simulink library "ammclib_bam_s32k14x"  (Simulink 9.0)
settings: Solver=ode45  StartTime=0.0  StopTime=10.0  RelTol=1e-3
undefined symbols (not defined in the file): f16A1, f16A2, f16B0, f16B1, f16B2, f16C1, f16CC1, f16CC1sc, f16CC1sc_D, f16CC1sc_Q, f16CC1scD, f16CC1scQ, f16CC2, f16CC2sc, f16CC2sc_D, f16CC2sc_Q, f16CC2scD, f16CC2scQ, f16DerivGain, f16EGain, f16FiltCoef, f16HystOff, f16HystOn, f16IGain, f16IntegGain, f16IntegGainFW, f16IntegGainQ, f16Kd, f16Kq, f16Limit, f16LowerLim, f16LowerLimit_D, f16LowerLimit_Q, f16ModIndex, f16OutValOff, f16OutValOn, f16PropGain, f16PropGainFW, f16PropGainQ, f16RampDown, f16RampUp, f16UGain, f16UpperLim, f16UpperLimit, f16UpperLimit_D, f16UpperLimit_Q, f16WIGain, f32A1, f32A2, f32B0, f32B1, f32B2, f32C1, f32CC1, f32CC1sc, f32CC1sc_D, f32CC1sc_Q, f32CC1scD, f32CC1scQ, f32CC2 ... (+122)
(part 8 of 11)

== system ammclib_bam_s32k14x/GMCLIB/bam_f32/GMCLIB_ClarkInv_F32 ==
  note: ---------------------------------------------------------------------------------------------------------------------------------------------------------------------------------------------------
  f32Alpha : Inport
  f32Beta : Inport  Port=2
  GMCLIB_ClarkInv_SF_F32 : S-Function  FunctionName=GMCLIB_ClarkInv_SF_F32  SFunctionDeploymentMode=off  EnableBusSupport=off
  copyright : Subsystem
      mask Display:
      | text(10,90,'FILE:');text(10,75,'DESRIPTION:')
      | text(10,60,'COPYRIGHT:')
      | text(10,45,'VERSION:')
      | text(10,30,'DATE:')
  copyright2 : Subsystem
      mask Display:
      | text(10,90,'GMCLIB_ClarkInv_BAM_F32.mdl');text(10,75,'Inverse Clarke transformation');text(10,60,'NXP')
      | text(10,45,'0.1');text(10,30,'30-Aug-2011');
  logo : Subsystem
      mask Display: image(imread('logo.jpg'))
  f32A : Outport
  f32B : Outport  Port=2
  f32C : Outport  Port=3
  wires:
  GMCLIB_ClarkInv_SF_F32/3 -> f32C/1
  GMCLIB_ClarkInv_SF_F32/2 -> f32B/1
  GMCLIB_ClarkInv_SF_F32/1 -> f32A/1
  f32Beta/1 -> GMCLIB_ClarkInv_SF_F32/2
  f32Alpha/1 -> GMCLIB_ClarkInv_SF_F32/1

== system ammclib_bam_s32k14x/GMCLIB/bam_f32/GMCLIB_Clark_F32 ==
  note: ---------------------------------------------------------------------------------------------------------------------------------------------------------------------------------------------------
  f32A : Inport
  f32B : Inport  Port=2
  f32C : Inport  Port=3
  GMCLIB_Clark_SF_F32 : S-Function  FunctionName=GMCLIB_Clark_SF_F32  SFunctionDeploymentMode=off  EnableBusSupport=off
  copyright : Subsystem
      mask Display:
      | text(10,90,'FILE:');text(10,75,'DESRIPTION:')
      | text(10,60,'COPYRIGHT:')
      | text(10,45,'VERSION:')
      | text(10,30,'DATE:')
  copyright2 : Subsystem
      mask Display:
      | text(10,90,'GMCLIB_Clark_BAM_F32.mdl');text(10,75,'Clarke transformation.');text(10,60,'NXP')
      | text(10,45,'0.1');text(10,30,'29-Aug-2011');
  logo : Subsystem
      mask Display: image(imread('logo.jpg'))
  f32Alpha : Outport
  f32Beta : Outport  Port=2
  wires:
  GMCLIB_Clark_SF_F32/2 -> f32Beta/1
  GMCLIB_Clark_SF_F32/1 -> f32Alpha/1
  f32C/1 -> GMCLIB_Clark_SF_F32/3
  f32B/1 -> GMCLIB_Clark_SF_F32/2
  f32A/1 -> GMCLIB_Clark_SF_F32/1

== system ammclib_bam_s32k14x/GMCLIB/bam_f32/GMCLIB_DecouplingPMSM_F32 ==
  note: ---------------------------------------------------------------------------------------------------------------------------------------------------------------------------------------------------
  f32Ud : Inport
  f32Uq : Inport  Port=2
  f32Id : Inport  Port=3
  f32Iq : Inport  Port=4
  f32AngVel : Inport  Port=5
  GMCLIB_DecouplingPMSM_SF_F32 : S-Function  FunctionName=GMCLIB_DecouplingPMSM_SF_F32  Parameters=f32Kd,s16KdShift,f32Kq,s16KqShift  SFunctionDeploymentMode=off  EnableBusSupport=off
  copyright : Subsystem
      mask Display:
      | text(10,90,'FILE:');text(10,75,'DESRIPTION:')
      | text(10,60,'COPYRIGHT:')
      | text(10,45,'VERSION:')
      | text(10,30,'DATE:')
  copyright2 : Subsystem
      mask Display:
      | text(10,90,'GMCLIB_DecouplingPMSM_BAM_F32.mdl');text(10,75,'Decoupling of d and q axis of PMSM model.');text(10,60,'NXP')
      | text(10,45,'0.1');text(10,30,'14-Sep-2011');
  logo : Subsystem
      mask Display: image(imread('logo.jpg'))
  f32UdDec : Outport
  f32UqDec : Outport  Port=2
  wires:
  GMCLIB_DecouplingPMSM_SF_F32/2 -> f32UqDec/1
  GMCLIB_DecouplingPMSM_SF_F32/1 -> f32UdDec/1
  f32AngVel/1 -> GMCLIB_DecouplingPMSM_SF_F32/5
  f32Iq/1 -> GMCLIB_DecouplingPMSM_SF_F32/4
  f32Id/1 -> GMCLIB_DecouplingPMSM_SF_F32/3
  f32Uq/1 -> GMCLIB_DecouplingPMSM_SF_F32/2
  f32Ud/1 -> GMCLIB_DecouplingPMSM_SF_F32/1

== system ammclib_bam_s32k14x/GMCLIB/bam_f32/GMCLIB_ElimDcBusRip_F32 ==
  note: ---------------------------------------------------------------------------------------------------------------------------------------------------------------------------------------------------
  f32Alpha : Inport
  f32Beta : Inport  Port=2
  f32ArgDcBusMsr : Inport  Port=3
  GMCLIB_ElimDcBusRip_SF : S-Function  FunctionName=GMCLIB_ElimDcBusRip_SF_F32  Parameters=f32ModIndex  SFunctionDeploymentMode=off  EnableBusSupport=off
  copyright : Subsystem
      mask Display: text(10,90,'FILE:');text(10,75,'DESRIPTION:');text(10,60,'COPYRIGHT:');text(10,45,'VERSION:');text(10,30,'DATE:')
  copyright2 : Subsystem
      mask Display: text(10,90,'GMCLIB_ElimDcBusRip_BAM_F32.mdl');text(10,75,'DC Bus voltage ripple elimination function.');text(10,60,'NXP');text(10,45,'0.1');text(10,30,'12-Jun-2015');
  logo : Subsystem
      mask Display: image(imread('logo.jpg'))
  f32AlphaOut : Outport
  f32BetaOut : Outport  Port=2
  wires:
  GMCLIB_ElimDcBusRip_SF/2 -> f32BetaOut/1
  GMCLIB_ElimDcBusRip_SF/1 -> f32AlphaOut/1
  f32ArgDcBusMsr/1 -> GMCLIB_ElimDcBusRip_SF/3
  f32Beta/1 -> GMCLIB_ElimDcBusRip_SF/2
  f32Alpha/1 -> GMCLIB_ElimDcBusRip_SF/1

== system ammclib_bam_s32k14x/GMCLIB/bam_f32/GMCLIB_ParkInv_F32 ==
  note: ---------------------------------------------------------------------------------------------------------------------------------------------------------------------------------------------------
  f32D : Inport
  f32Q : Inport  Port=2
  f32Sin : Inport  Port=3
  f32Cos : Inport  Port=4
  GMCLIB_ParkInv_SF : S-Function  FunctionName=GMCLIB_ParkInv_SF_F32  SFunctionDeploymentMode=off  EnableBusSupport=off
  copyright : Subsystem
      mask Display:
      | text(10,90,'FILE:');text(10,75,'DESRIPTION:')
      | text(10,60,'COPYRIGHT:')
      | text(10,45,'VERSION:')
      | text(10,30,'DATE:')
  copyright2 : Subsystem
      mask Display:
      | text(10,90,'GMCLIB_ParkInv_BAM_F32.mdl');text(10,75,'Inverse Park transformation.');text(10,60,'Freescale')
      | text(10,45,'0.1');text(10,30,'19-Sep-2011');
  logo : Subsystem
      mask Display: image(imread('logo.jpg'))
  f32Alpha : Outport
  f32Beta : Outport  Port=2
  wires:
  GMCLIB_ParkInv_SF/2 -> f32Beta/1
  GMCLIB_ParkInv_SF/1 -> f32Alpha/1
  f32Cos/1 -> GMCLIB_ParkInv_SF/4
  f32Sin/1 -> GMCLIB_ParkInv_SF/3
  f32Q/1 -> GMCLIB_ParkInv_SF/2
  f32D/1 -> GMCLIB_ParkInv_SF/1

== system ammclib_bam_s32k14x/GMCLIB/bam_f32/GMCLIB_Park_F32 ==
  note: ---------------------------------------------------------------------------------------------------------------------------------------------------------------------------------------------------
  f32Alpha : Inport
  f32Beta : Inport  Port=2
  f32Sin : Inport  Port=3
  f32Cos : Inport  Port=4
  GMCLIB_Park_SF : S-Function  FunctionName=GMCLIB_Park_SF_F32  SFunctionDeploymentMode=off  EnableBusSupport=off
  copyright : Subsystem
      mask Display:
      | text(10,90,'FILE:');text(10,75,'DESRIPTION:')
      | text(10,60,'COPYRIGHT:')
      | text(10,45,'VERSION:')
      | text(10,30,'DATE:')
  copyright2 : Subsystem
      mask Display:
      | text(10,90,'GMCLIB_Park_BAM_F32.mdl');text(10,75,'Park transformation.');text(10,60,'NXP')
      | text(10,45,'0.1');text(10,30,'19-Sep-2011');
  logo : Subsystem
      mask Display: image(imread('logo.jpg'))
  f32D : Outport
  f32Q : Outport  Port=2
  wires:
  GMCLIB_Park_SF/2 -> f32Q/1
  GMCLIB_Park_SF/1 -> f32D/1
  f32Cos/1 -> GMCLIB_Park_SF/4
  f32Sin/1 -> GMCLIB_Park_SF/3
  f32Beta/1 -> GMCLIB_Park_SF/2
  f32Alpha/1 -> GMCLIB_Park_SF/1

== system ammclib_bam_s32k14x/GMCLIB/bam_f32/GMCLIB_PwmIct_F32 ==
  note: ---------------------------------------------------------------------------------------------------------------------------------------------------------------------------------------------------
  f32In1 : Inport
  f32In2 : Inport  Port=2
  GMCLIB_PwmIct_SF : S-Function  FunctionName=GMCLIB_PwmIct_SF_F32  SFunctionDeploymentMode=off  EnableBusSupport=off
  copyright : Subsystem
      mask Display: text(10,90,'FILE:');text(10,75,'DESRIPTION:');text(10,60,'COPYRIGHT:');text(10,45,'VERSION:');text(10,30,'DATE:')
  copyright2 : Subsystem
      mask Display: text(10,90,'GMCLIB_PwmIct_BAM_F32.mdl');text(10,75,'General Sinusoidal PWM.');text(10,60,'NXP');text(10,45,'1.0');text(10,30,'05-Apr-2019');
  logo : Subsystem
      mask Display: image(imread('logo.jpg'))
  f32Out1 : Outport
  f32Out2 : Outport  Port=2
  f32Out3 : Outport  Port=3
  u32Sector : Outport  Port=4
  wires:
  f32In1/1 -> GMCLIB_PwmIct_SF/1
  f32In2/1 -> GMCLIB_PwmIct_SF/2
  GMCLIB_PwmIct_SF/1 -> f32Out1/1
  GMCLIB_PwmIct_SF/2 -> f32Out2/1
  GMCLIB_PwmIct_SF/3 -> f32Out3/1
  GMCLIB_PwmIct_SF/4 -> u32Sector/1

== system ammclib_bam_s32k14x/GMCLIB/bam_f32/GMCLIB_SvmStd_F32 ==
  note: ---------------------------------------------------------------------------------------------------------------------------------------------------------------------------------------------------
  f32In1 : Inport
  f32In2 : Inport  Port=2
  GMCLIB_SvmStd_SF : S-Function  FunctionName=GMCLIB_SvmStd_SF_F32  SFunctionDeploymentMode=off  EnableBusSupport=off
  copyright : Subsystem
      mask Display:
      | text(10,90,'FILE:');text(10,75,'DESRIPTION:')
      | text(10,60,'COPYRIGHT:')
      | text(10,45,'VERSION:')
      | text(10,30,'DATE:')
  copyright2 : Subsystem
      mask Display:
      | text(10,90,'GMCLIB_SvmStd_BAM_F32.mdl');text(10,75,'Standard Space Vector Modulation.');text(10,60,'NXP')
      | text(10,45,'0.1');text(10,30,'26-Sep-2011');
  logo : Subsystem
      mask Display: image(imread('logo.jpg'))
  f32Out1 : Outport
  f32Out2 : Outport  Port=2
  f32Out3 : Outport  Port=3
  u32Sector : Outport  Port=4
  wires:
  GMCLIB_SvmStd_SF/4 -> u32Sector/1
  GMCLIB_SvmStd_SF/3 -> f32Out3/1
  GMCLIB_SvmStd_SF/2 -> f32Out2/1
  GMCLIB_SvmStd_SF/1 -> f32Out1/1
  f32In2/1 -> GMCLIB_SvmStd_SF/2
  f32In1/1 -> GMCLIB_SvmStd_SF/1

== system ammclib_bam_s32k14x/GMCLIB/bam_f32/GMCLIB_SvmU0n_F32 ==
  note: ---------------------------------------------------------------------------------------------------------------------------------------------------------------------------------------------------
  f32In1 : Inport
  f32In2 : Inport  Port=2
  GMCLIB_SvmU0n_SF : S-Function  FunctionName=GMCLIB_SvmU0n_SF_F32  SFunctionDeploymentMode=off  EnableBusSupport=off
  copyright : Subsystem
      mask Display: text(10,90,'FILE:');text(10,75,'DESRIPTION:');text(10,60,'COPYRIGHT:');text(10,45,'VERSION:');text(10,30,'DATE:')
  copyright2 : Subsystem
      mask Display: text(10,90,'GMCLIB_SvmU0n_BAM_F32.mdl');text(10,75,'Standard Space Vector Modulation.');text(10,60,'NXP');text(10,45,'0.1');text(10,30,'02-Apr-2019');
  logo : Subsystem
      mask Display: image(imread('logo.jpg'))
  f32Out1 : Outport
  f32Out2 : Outport  Port=2
  f32Out3 : Outport  Port=3
  u32Sector : Outport  Port=4
  wires:
  f32In1/1 -> GMCLIB_SvmU0n_SF/1
  f32In2/1 -> GMCLIB_SvmU0n_SF/2
  GMCLIB_SvmU0n_SF/1 -> f32Out1/1
  GMCLIB_SvmU0n_SF/2 -> f32Out2/1
  GMCLIB_SvmU0n_SF/3 -> f32Out3/1
  GMCLIB_SvmU0n_SF/4 -> u32Sector/1

== system ammclib_bam_s32k14x/GMCLIB/bam_flt/GMCLIB_ClarkInv_FLT ==
  note: ---------------------------------------------------------------------------------------------------------------------------------------------------------------------------------------------------
  fltAlpha : Inport
  fltBeta : Inport  Port=2
  GMCLIB_ClarkInv_SF_FLT : S-Function  FunctionName=GMCLIB_ClarkInv_SF_FLT  SFunctionDeploymentMode=off  EnableBusSupport=off
  copyright : Subsystem
      mask Display:
      | text(10,90,'FILE:');text(10,75,'DESRIPTION:')
      | text(10,60,'COPYRIGHT:')
      | text(10,45,'VERSION:')
      | text(10,30,'DATE:')
  copyright2 : Subsystem
      mask Display:
      | text(10,90,'GMCLIB_ClarkInv_BAM_FLT.mdl');text(10,75,'Inverse Clarke transformation');text(10,60,'NXP')
      | text(10,45,'0.1');text(10,30,'30-Aug-2011');
  logo : Subsystem
      mask Display: image(imread('logo.jpg'))
  fltA : Outport
  fltB : Outport  Port=2
  fltC : Outport  Port=3
  wires:
  GMCLIB_ClarkInv_SF_FLT/3 -> fltC/1
  GMCLIB_ClarkInv_SF_FLT/2 -> fltB/1
  GMCLIB_ClarkInv_SF_FLT/1 -> fltA/1
  fltBeta/1 -> GMCLIB_ClarkInv_SF_FLT/2
  fltAlpha/1 -> GMCLIB_ClarkInv_SF_FLT/1

== system ammclib_bam_s32k14x/GMCLIB/bam_flt/GMCLIB_Clark_FLT ==
  note: ---------------------------------------------------------------------------------------------------------------------------------------------------------------------------------------------------
  fltA : Inport
  fltB : Inport  Port=2
  fltC : Inport  Port=3
  GMCLIB_Clark_SF_FLT : S-Function  FunctionName=GMCLIB_Clark_SF_FLT  SFunctionDeploymentMode=off  EnableBusSupport=off
  copyright : Subsystem
      mask Display:
      | text(10,90,'FILE:');text(10,75,'DESRIPTION:')
      | text(10,60,'COPYRIGHT:')
      | text(10,45,'VERSION:')
      | text(10,30,'DATE:')
  copyright2 : Subsystem
      mask Display:
      | text(10,90,'GMCLIB_Clark_BAM_FLT.mdl');text(10,75,'Clarke transformation.');text(10,60,'NXP')
      | text(10,45,'0.1');text(10,30,'29-Aug-2011');
  logo : Subsystem
      mask Display: image(imread('logo.jpg'))
  fltAlpha : Outport
  fltBeta : Outport  Port=2
  wires:
  GMCLIB_Clark_SF_FLT/2 -> fltBeta/1
  GMCLIB_Clark_SF_FLT/1 -> fltAlpha/1
  fltC/1 -> GMCLIB_Clark_SF_FLT/3
  fltB/1 -> GMCLIB_Clark_SF_FLT/2
  fltA/1 -> GMCLIB_Clark_SF_FLT/1

== system ammclib_bam_s32k14x/GMCLIB/bam_flt/GMCLIB_DecouplingPMSM_FLT ==
  note: ---------------------------------------------------------------------------------------------------------------------------------------------------------------------------------------------------
  fltUd : Inport
  fltUq : Inport  Port=2
  fltId : Inport  Port=3
  fltIq : Inport  Port=4
  fltAngVel : Inport  Port=5
  GMCLIB_DecouplingPMSM_SF_FLT : S-Function  FunctionName=GMCLIB_DecouplingPMSM_SF_FLT  Parameters=fltKd,fltKq  SFunctionDeploymentMode=off  EnableBusSupport=off
  copyright : Subsystem
      mask Display:
      | text(10,90,'FILE:');text(10,75,'DESRIPTION:')
      | text(10,60,'COPYRIGHT:')
      | text(10,45,'VERSION:')
      | text(10,30,'DATE:')
  copyright2 : Subsystem
      mask Display:
      | text(10,90,'GMCLIB_DecouplingPMSM_BAM_FLT.mdl');text(10,75,'Decoupling of d and q axis of PMSM model.');text(10,60,'NXP')
      | text(10,45,'0.1');text(10,30,'14-Sep-2011');
  logo : Subsystem
      mask Display: image(imread('logo.jpg'))
  fltUdDec : Outport
  fltUqDec : Outport  Port=2
  wires:
  GMCLIB_DecouplingPMSM_SF_FLT/2 -> fltUqDec/1
  GMCLIB_DecouplingPMSM_SF_FLT/1 -> fltUdDec/1
  fltAngVel/1 -> GMCLIB_DecouplingPMSM_SF_FLT/5
  fltIq/1 -> GMCLIB_DecouplingPMSM_SF_FLT/4
  fltId/1 -> GMCLIB_DecouplingPMSM_SF_FLT/3
  fltUq/1 -> GMCLIB_DecouplingPMSM_SF_FLT/2
  fltUd/1 -> GMCLIB_DecouplingPMSM_SF_FLT/1

== system ammclib_bam_s32k14x/GMCLIB/bam_flt/GMCLIB_ElimDcBusRip_FLT ==
  note: ---------------------------------------------------------------------------------------------------------------------------------------------------------------------------------------------------
  fltAlpha : Inport
  fltBeta : Inport  Port=2
  fltArgDcBusMsr : Inport  Port=3
  GMCLIB_ElimDcBusRip_SF : S-Function  FunctionName=GMCLIB_ElimDcBusRip_SF_FLT  Parameters=fltModIndex  SFunctionDeploymentMode=off  EnableBusSupport=off
  copyright : Subsystem
      mask Display: text(10,90,'FILE:');text(10,75,'DESRIPTION:');text(10,60,'COPYRIGHT:');text(10,45,'VERSION:');text(10,30,'DATE:')
  copyright2 : Subsystem
      mask Display: text(10,90,'GMCLIB_ElimDcBusRip_BAM_FLT.mdl');text(10,75,'DC Bus voltage ripple elimination function.');text(10,60,'NXP');text(10,45,'0.1');text(10,30,'12-Jun-2015');
  logo : Subsystem
      mask Display: image(imread('logo.jpg'))
  fltAlphaOut : Outport
  fltBetaOut : Outport  Port=2
  wires:
  GMCLIB_ElimDcBusRip_SF/2 -> fltBetaOut/1
  GMCLIB_ElimDcBusRip_SF/1 -> fltAlphaOut/1
  fltArgDcBusMsr/1 -> GMCLIB_ElimDcBusRip_SF/3
  fltBeta/1 -> GMCLIB_ElimDcBusRip_SF/2
  fltAlpha/1 -> GMCLIB_ElimDcBusRip_SF/1

== system ammclib_bam_s32k14x/GMCLIB/bam_flt/GMCLIB_ParkInv_FLT ==
  note: ---------------------------------------------------------------------------------------------------------------------------------------------------------------------------------------------------
  fltD : Inport
  fltQ : Inport  Port=2
  fltSin : Inport  Port=3
  fltCos : Inport  Port=4
  GMCLIB_ParkInv_SF : S-Function  FunctionName=GMCLIB_ParkInv_SF_FLT  SFunctionDeploymentMode=off  EnableBusSupport=off
  copyright : Subsystem
      mask Display:
      | text(10,90,'FILE:');text(10,75,'DESRIPTION:')
      | text(10,60,'COPYRIGHT:')
      | text(10,45,'VERSION:')
      | text(10,30,'DATE:')
  copyright2 : Subsystem
      mask Display:
      | text(10,90,'GMCLIB_ParkInv_BAM_FLT.mdl');text(10,75,'Inverse Park transformation.');text(10,60,'Freescale')
      | text(10,45,'0.1');text(10,30,'19-Sep-2011');
  logo : Subsystem
      mask Display: image(imread('logo.jpg'))
  fltAlpha : Outport
  fltBeta : Outport  Port=2
  wires:
  GMCLIB_ParkInv_SF/2 -> fltBeta/1
  GMCLIB_ParkInv_SF/1 -> fltAlpha/1
  fltCos/1 -> GMCLIB_ParkInv_SF/4
  fltSin/1 -> GMCLIB_ParkInv_SF/3
  fltQ/1 -> GMCLIB_ParkInv_SF/2
  fltD/1 -> GMCLIB_ParkInv_SF/1

== system ammclib_bam_s32k14x/GMCLIB/bam_flt/GMCLIB_Park_FLT ==
  note: ---------------------------------------------------------------------------------------------------------------------------------------------------------------------------------------------------
  fltAlpha : Inport
  fltBeta : Inport  Port=2
  fltSin : Inport  Port=3
  fltCos : Inport  Port=4
  GMCLIB_Park_SF : S-Function  FunctionName=GMCLIB_Park_SF_FLT  SFunctionDeploymentMode=off  EnableBusSupport=off
  copyright : Subsystem
      mask Display:
      | text(10,90,'FILE:');text(10,75,'DESRIPTION:')
      | text(10,60,'COPYRIGHT:')
      | text(10,45,'VERSION:')
      | text(10,30,'DATE:')
  copyright2 : Subsystem
      mask Display:
      | text(10,90,'GMCLIB_Park_BAM_FLT.mdl');text(10,75,'Park transformation.');text(10,60,'NXP')
      | text(10,45,'0.1');text(10,30,'19-Sep-2011');
  logo : Subsystem
      mask Display: image(imread('logo.jpg'))
  fltD : Outport
  fltQ : Outport  Port=2
  wires:
  GMCLIB_Park_SF/2 -> fltQ/1
  GMCLIB_Park_SF/1 -> fltD/1
  fltCos/1 -> GMCLIB_Park_SF/4
  fltSin/1 -> GMCLIB_Park_SF/3
  fltBeta/1 -> GMCLIB_Park_SF/2
  fltAlpha/1 -> GMCLIB_Park_SF/1

== system ammclib_bam_s32k14x/GMCLIB/bam_flt/GMCLIB_PwmIct_FLT ==
  note: ---------------------------------------------------------------------------------------------------------------------------------------------------------------------------------------------------
  fltIn1 : Inport
  fltIn2 : Inport  Port=2
  GMCLIB_PwmIct_SF : S-Function  FunctionName=GMCLIB_PwmIct_SF_FLT  SFunctionDeploymentMode=off  EnableBusSupport=off
  copyright : Subsystem
      mask Display: text(10,90,'FILE:');text(10,75,'DESRIPTION:');text(10,60,'COPYRIGHT:');text(10,45,'VERSION:');text(10,30,'DATE:')
  copyright2 : Subsystem
      mask Display: text(10,90,'GMCLIB_PwmIct_BAM_FLT.mdl');text(10,75,'General Sinusoidal PWM.');text(10,60,'NXP');text(10,45,'1.0');text(10,30,'05-Apr-2019');
  logo : Subsystem
      mask Display: image(imread('logo.jpg'))
  fltOut1 : Outport
  fltOut2 : Outport  Port=2
  fltOut3 : Outport  Port=3
  u32Sector : Outport  Port=4
  wires:
  fltIn1/1 -> GMCLIB_PwmIct_SF/1
  fltIn2/1 -> GMCLIB_PwmIct_SF/2
  GMCLIB_PwmIct_SF/1 -> fltOut1/1
  GMCLIB_PwmIct_SF/2 -> fltOut2/1
  GMCLIB_PwmIct_SF/3 -> fltOut3/1
  GMCLIB_PwmIct_SF/4 -> u32Sector/1

== system ammclib_bam_s32k14x/GMCLIB/bam_flt/GMCLIB_SvmStd_FLT ==
  note: ---------------------------------------------------------------------------------------------------------------------------------------------------------------------------------------------------
  fltIn1 : Inport
  fltIn2 : Inport  Port=2
  GMCLIB_SvmStd_SF : S-Function  FunctionName=GMCLIB_SvmStd_SF_FLT  SFunctionDeploymentMode=off  EnableBusSupport=off
  copyright : Subsystem
      mask Display:
      | text(10,90,'FILE:');text(10,75,'DESRIPTION:')
      | text(10,60,'COPYRIGHT:')
      | text(10,45,'VERSION:')
      | text(10,30,'DATE:')
  copyright2 : Subsystem
      mask Display:
      | text(10,90,'GMCLIB_SvmStd_BAM_FLT.mdl');text(10,75,'Standard Space Vector Modulation.');text(10,60,'NXP')
      | text(10,45,'0.1');text(10,30,'26-Sep-2011');
  logo : Subsystem
      mask Display: image(imread('logo.jpg'))
  fltOut1 : Outport
  fltOut2 : Outport  Port=2
  fltOut3 : Outport  Port=3
  u32Sector : Outport  Port=4
  wires:
  GMCLIB_SvmStd_SF/4 -> u32Sector/1
  GMCLIB_SvmStd_SF/3 -> fltOut3/1
  GMCLIB_SvmStd_SF/2 -> fltOut2/1
  GMCLIB_SvmStd_SF/1 -> fltOut1/1
  fltIn2/1 -> GMCLIB_SvmStd_SF/2
  fltIn1/1 -> GMCLIB_SvmStd_SF/1

== system ammclib_bam_s32k14x/GMCLIB/bam_flt/GMCLIB_SvmU0n_FLT ==
  note: ---------------------------------------------------------------------------------------------------------------------------------------------------------------------------------------------------
  fltIn1 : Inport
  fltIn2 : Inport  Port=2
  GMCLIB_SvmU0n_SF : S-Function  FunctionName=GMCLIB_SvmU0n_SF_FLT  SFunctionDeploymentMode=off  EnableBusSupport=off
  copyright : Subsystem
      mask Display: text(10,90,'FILE:');text(10,75,'DESRIPTION:');text(10,60,'COPYRIGHT:');text(10,45,'VERSION:');text(10,30,'DATE:')
  copyright2 : Subsystem
      mask Display: text(10,90,'GMCLIB_SvmU0n_BAM_FLT.mdl');text(10,75,'Standard Space Vector Modulation.');text(10,60,'NXP');text(10,45,'0.1');text(10,30,'02-Apr-2019');
  logo : Subsystem
      mask Display: image(imread('logo.jpg'))
  fltOut1 : Outport
  fltOut2 : Outport  Port=2
  fltOut3 : Outport  Port=3
  u32Sector : Outport  Port=4
  wires:
  fltIn1/1 -> GMCLIB_SvmU0n_SF/1
  fltIn2/1 -> GMCLIB_SvmU0n_SF/2
  GMCLIB_SvmU0n_SF/1 -> fltOut1/1
  GMCLIB_SvmU0n_SF/2 -> fltOut2/1
  GMCLIB_SvmU0n_SF/3 -> fltOut3/1
  GMCLIB_SvmU0n_SF/4 -> u32Sector/1

== system ammclib_bam_s32k14x/MLIB/bam_f16/MLIB_AbsSat_F16 ==
  note: ---------------------------------------------------------------------------------------------------------------------------------------------------------------------------------------------------
  f16In : Inport
  MLIB_AbsSat_SF : S-Function  FunctionName=MLIB_AbsSat_SF_F16  SFunctionDeploymentMode=off  EnableBusSupport=off
  copyright : Subsystem
      mask Display:
      | text(10,90,'FILE:');text(10,75,'DESRIPTION:')
      | text(10,60,'COPYRIGHT:')
      | text(10,45,'VERSION:')
      | text(10,30,'DATE:')
  copyright2 : Subsystem
      mask Display:
      | text(10,90,'MLIB_AbsSat_BAM_F16.mdl');text(10,75,'Absolute value of input parameter saturated if necessary.');text(10,60,'NXP')
      | text(10,45,'0.1');text(10,30,'19-Aug-2011');
  logo : Subsystem
      mask Display: image(imread('logo.jpg'))
  f16Out : Outport
  wires:
  MLIB_AbsSat_SF/1 -> f16Out/1
  f16In/1 -> MLIB_AbsSat_SF/1

== system ammclib_bam_s32k14x/MLIB/bam_f16/MLIB_Abs_F16 ==
  note: ---------------------------------------------------------------------------------------------------------------------------------------------------------------------------------------------------
  f16In : Inport
  MLIB_Abs_SF : S-Function  FunctionName=MLIB_Abs_SF_F16  SFunctionDeploymentMode=off  EnableBusSupport=off
  copyright : Subsystem
      mask Display:
      | text(10,90,'FILE:');text(10,75,'DESRIPTION:')
      | text(10,60,'COPYRIGHT:')
      | text(10,45,'VERSION:')
      | text(10,30,'DATE:')
  copyright2 : Subsystem
      mask Display:
      | text(10,90,'MLIB_Abs_BAM_F16.mdl');text(10,75,'Absolute value of input parameter.');text(10,60,'Freescale')
      | text(10,45,'0.1');text(10,30,'20-Jan-2012');
  logo : Subsystem
      mask Display: image(imread('logo.jpg'))
  f16Out : Outport
  wires:
  MLIB_Abs_SF/1 -> f16Out/1
  f16In/1 -> MLIB_Abs_SF/1

== system ammclib_bam_s32k14x/MLIB/bam_f16/MLIB_AddSat_F16 ==
  note: ---------------------------------------------------------------------------------------------------------------------------------------------------------------------------------------------------
  f16In1 : Inport
  f16In2 : Inport  Port=2
  MLIB_AddSat_SF : S-Function  FunctionName=MLIB_AddSat_SF_F16  SFunctionDeploymentMode=off  EnableBusSupport=off
  copyright : Subsystem
      mask Display:
      | text(10,90,'FILE:');text(10,75,'DESRIPTION:')
      | text(10,60,'COPYRIGHT:')
      | text(10,45,'VERSION:')
      | text(10,30,'DATE:')
  copyright2 : Subsystem
      mask Display:
      | text(10,90,'MLIB_AddSat_BAM_F16.mdl');text(10,75,'Saturated sum of two input values.');text(10,60,'NXP')
      | text(10,45,'0.1');text(10,30,'20-Jan-2012');
  logo : Subsystem
      mask Display: image(imread('logo.jpg'))
  f16Out : Outport
  wires:
  MLIB_AddSat_SF/1 -> f16Out/1
  f16In2/1 -> MLIB_AddSat_SF/2
  f16In1/1 -> MLIB_AddSat_SF/1

== system ammclib_bam_s32k14x/MLIB/bam_f16/MLIB_Add_F16 ==
  note: ---------------------------------------------------------------------------------------------------------------------------------------------------------------------------------------------------
  f16In1 : Inport
  f16In2 : Inport  Port=2
  MLIB_Add_SF : S-Function  FunctionName=MLIB_Add_SF_F16  SFunctionDeploymentMode=off  EnableBusSupport=off
  copyright : Subsystem
      mask Display:
      | text(10,90,'FILE:');text(10,75,'DESRIPTION:')
      | text(10,60,'COPYRIGHT:')
      | text(10,45,'VERSION:')
      | text(10,30,'DATE:')
  copyright2 : Subsystem
      mask Display:
      | text(10,90,'MLIB_Add_BAM_F16.mdl');text(10,75,'Sum of two input values.');text(10,60,'NXP')
      | text(10,45,'0.1');text(10,30,'20-Jan-2012');
  logo : Subsystem
      mask Display: image(imread('logo.jpg'))
  f16Out : Outport
  wires:
  MLIB_Add_SF/1 -> f16Out/1
  f16In2/1 -> MLIB_Add_SF/2
  f16In1/1 -> MLIB_Add_SF/1

== system ammclib_bam_s32k14x/MLIB/bam_f16/MLIB_ConvertPU_F16F32 ==
  note: ---------------------------------------------------------------------------------------------------------------------------------------------------------------------------------------------------
  f32In : Inport
  MLIB_ConvertPU_SF : S-Function  FunctionName=MLIB_ConvertPU_SF_F16F32  SFunctionDeploymentMode=off  EnableBusSupport=off
  copyright : Subsystem
      mask Display:
      | text(10,90,'FILE:');text(10,75,'DESRIPTION:')
      | text(10,60,'COPYRIGHT:')
      | text(10,45,'VERSION:')
      | text(10,30,'DATE:')
  copyright2 : Subsystem
      mask Display:
      | text(10,90,'MLIB_ConvertPU_BAM_F16.mdl');text(10,75,'Converts the input value to different representation in unity model.');text(10,60,'NXP')
      | text(10,45,'0.1');text(10,30,'10-Oct-2011');
  logo : Subsystem
      mask Display: image(imread('logo.jpg'))
  f16Out : Outport
  wires:
  MLIB_ConvertPU_SF/1 -> f16Out/1
  f32In/1 -> MLIB_ConvertPU_SF/1

== system ammclib_bam_s32k14x/MLIB/bam_f16/MLIB_ConvertPU_F16FLT ==
  note: ---------------------------------------------------------------------------------------------------------------------------------------------------------------------------------------------------
  fltIn : Inport
  MLIB_ConvertPU_SF : S-Function  FunctionName=MLIB_ConvertPU_SF_F16FLT  SFunctionDeploymentMode=off  EnableBusSupport=off
  copyright : Subsystem
      mask Display:
      | text(10,90,'FILE:');text(10,75,'DESRIPTION:')
      | text(10,60,'COPYRIGHT:')
      | text(10,45,'VERSION:')
      | text(10,30,'DATE:')
  copyright2 : Subsystem
      mask Display:
      | text(10,90,'MLIB_ConvertPU_BAM_F16.mdl');text(10,75,'Converts the input value to different representation in unity model.');text(10,60,'NXP')
      | text(10,45,'0.1');text(10,30,'10-Oct-2011');
  logo : Subsystem
      mask Display: image(imread('logo.jpg'))
  f16Out : Outport
  wires:
  MLIB_ConvertPU_SF/1 -> f16Out/1
  fltIn/1 -> MLIB_ConvertPU_SF/1

== system ammclib_bam_s32k14x/MLIB/bam_f16/MLIB_Convert_F16F32 ==
  note: ---------------------------------------------------------------------------------------------------------------------------------------------------------------------------------------------------
  f32In1 : Inport
  f32In2 : Inport  Port=2
  MLIB_Convert_SF : S-Function  FunctionName=MLIB_Convert_SF_F16F32  SFunctionDeploymentMode=off  EnableBusSupport=off
  copyright : Subsystem
      mask Display:
      | text(10,90,'FILE:');text(10,75,'DESRIPTION:')
      | text(10,60,'COPYRIGHT:')
      | text(10,45,'VERSION:')
      | text(10,30,'DATE:')
  copyright2 : Subsystem
      mask Display:
      | text(10,90,'MLIB_Convert_BAM_F16F32.mdl');text(10,75,'Converts the input value with scale to different representation in unity model.');text(10,60,'NXP')
      | text(10,45,'0.1');text(10,30,'13-Oct-2011');
  logo : Subsystem
      mask Display: image(imread('logo.jpg'))
  f16Out : Outport
  wires:
  MLIB_Convert_SF/1 -> f16Out/1
  f32In2/1 -> MLIB_Convert_SF/2
  f32In1/1 -> MLIB_Convert_SF/1

== system ammclib_bam_s32k14x/MLIB/bam_f16/MLIB_Convert_F16FLT ==
  note: ---------------------------------------------------------------------------------------------------------------------------------------------------------------------------------------------------
  fltIn1 : Inport
  fltIn2 : Inport  Port=2
  MLIB_Convert_SF : S-Function  FunctionName=MLIB_Convert_SF_F16FLT  SFunctionDeploymentMode=off  EnableBusSupport=off
  copyright : Subsystem
      mask Display:
      | text(10,90,'FILE:');text(10,75,'DESRIPTION:')
      | text(10,60,'COPYRIGHT:')
      | text(10,45,'VERSION:')
      | text(10,30,'DATE:')
  copyright2 : Subsystem
      mask Display:
      | text(10,90,'MLIB_Convert_BAM_F16FLT.mdl');text(10,75,'Converts the input value with scale to different representation in unity model.');text(10,60,'NXP')
      | text(10,45,'0.1');text(10,30,'13-Oct-2011');
  logo : Subsystem
      mask Display: image(imread('logo.jpg'))
  f16Out : Outport
  wires:
  MLIB_Convert_SF/1 -> f16Out/1
  fltIn2/1 -> MLIB_Convert_SF/2
  fltIn1/1 -> MLIB_Convert_SF/1

== system ammclib_bam_s32k14x/MLIB/bam_f16/MLIB_DivSat_F16 ==
  note: ---------------------------------------------------------------------------------------------------------------------------------------------------------------------------------------------------
  f16In1 : Inport
  f16In2 : Inport  Port=2
  MLIB_DivSat_SF : S-Function  FunctionName=MLIB_DivSat_SF_F16  SFunctionDeploymentMode=off  EnableBusSupport=off
  copyright : Subsystem
      mask Display:
      | text(10,90,'FILE:');text(10,75,'DESRIPTION:')
      | text(10,60,'COPYRIGHT:')
      | text(10,45,'VERSION:')
      | text(10,30,'DATE:')
  copyright2 : Subsystem
      mask Display:
      | text(10,90,'MLIB_DivSat_BAM_F16.mdl');text(10,75,'Division of two input values saturated if necessary.');text(10,60,'NXP')
      | text(10,45,'0.1');text(10,30,'19-Aug-2011');
  logo : Subsystem
      mask Display: image(imread('logo.jpg'))
  f16Out : Outport
  wires:
  MLIB_DivSat_SF/1 -> f16Out/1
  f16In2/1 -> MLIB_DivSat_SF/2
  f16In1/1 -> MLIB_DivSat_SF/1

== system ammclib_bam_s32k14x/MLIB/bam_f16/MLIB_Div_F16 ==
  note: ---------------------------------------------------------------------------------------------------------------------------------------------------------------------------------------------------
  f16In1 : Inport
  f16In2 : Inport  Port=2
  MLIB_Div_SF : S-Function  FunctionName=MLIB_Div_SF_F16  SFunctionDeploymentMode=off  EnableBusSupport=off
  copyright : Subsystem
      mask Display:
      | text(10,90,'FILE:');text(10,75,'DESRIPTION:')
      | text(10,60,'COPYRIGHT:')
      | text(10,45,'VERSION:')
      | text(10,30,'DATE:')
  copyright2 : Subsystem
      mask Display:
      | text(10,90,'MLIB_Div_BAM_F16.mdl');text(10,75,'Division of two input values.');text(10,60,'Freescale')
      | text(10,45,'0.1');text(10,30,'19-Aug-2011');
  logo : Subsystem
      mask Display: image(imread('logo.jpg'))
  f16Out : Outport
  wires:
  MLIB_Div_SF/1 -> f16Out/1
  f16In2/1 -> MLIB_Div_SF/2
  f16In1/1 -> MLIB_Div_SF/1

== system ammclib_bam_s32k14x/MLIB/bam_f16/MLIB_MacSat_F16 ==
  note: ---------------------------------------------------------------------------------------------------------------------------------------------------------------------------------------------------
  f16In1 : Inport
  f16In2 : Inport  Port=2
  f16In3 : Inport  Port=3
  MLIB_MacSat_SF : S-Function  FunctionName=MLIB_MacSat_SF_F16  SFunctionDeploymentMode=off  EnableBusSupport=off
  copyright : Subsystem
      mask Display:
      | text(10,90,'FILE:');text(10,75,'DESRIPTION:')
      | text(10,60,'COPYRIGHT:')
      | text(10,45,'VERSION:')
      | text(10,30,'DATE:')
  copyright2 : Subsystem
      mask Display:
      | text(10,90,'MLIB_MacSat_BAM_F16.mdl');text(10,75,'Saturated sum of two input values.');text(10,60,'NXP')
      | text(10,45,'0.1');text(10,30,'22-Aug-2011');
  logo : Subsystem
      mask Display: image(imread('logo.jpg'))
  f16Out : Outport
  wires:
  MLIB_MacSat_SF/1 -> f16Out/1
  f16In3/1 -> MLIB_MacSat_SF/3
  f16In2/1 -> MLIB_MacSat_SF/2
  f16In1/1 -> MLIB_MacSat_SF/1

== system ammclib_bam_s32k14x/MLIB/bam_f16/MLIB_Mac_F16 ==
  note: ---------------------------------------------------------------------------------------------------------------------------------------------------------------------------------------------------
  f16In1 : Inport
  f16In2 : Inport  Port=2
  f16In3 : Inport  Port=3
  MLIB_Mac_SF : S-Function  FunctionName=MLIB_Mac_SF_F16  SFunctionDeploymentMode=off  EnableBusSupport=off
  copyright : Subsystem
      mask Display:
      | text(10,90,'FILE:');text(10,75,'DESRIPTION:')
      | text(10,60,'COPYRIGHT:')
      | text(10,45,'VERSION:')
      | text(10,30,'DATE:')
  copyright2 : Subsystem
      mask Display:
      | text(10,90,'MLIB_Mac_BAM_F16.mdl');text(10,75,'Sum of two input values.');text(10,60,'NXP')
      | text(10,45,'0.1');text(10,30,'18-Jul-2011');
  logo : Subsystem
      mask Display: image(imread('logo.jpg'))
  f16Out : Outport
  wires:
  MLIB_Mac_SF/1 -> f16Out/1
  f16In3/1 -> MLIB_Mac_SF/3
  f16In2/1 -> MLIB_Mac_SF/2
  f16In1/1 -> MLIB_Mac_SF/1

== system ammclib_bam_s32k14x/MLIB/bam_f16/MLIB_Mnac_F16 ==
  note: ---------------------------------------------------------------------------------------------------------------------------------------------------------------------------------------------------
  f16In1 : Inport
  f16In2 : Inport  Port=2
  f16In3 : Inport  Port=3
  MLIB_Mnac_SF : S-Function  FunctionName=MLIB_Mnac_SF_F16  SFunctionDeploymentMode=off  EnableBusSupport=off
  copyright : Subsystem
      mask Display:
      | text(10,90,'FILE:');text(10,75,'DESRIPTION:')
      | text(10,60,'COPYRIGHT:')
      | text(10,45,'VERSION:')
      | text(10,30,'DATE:')
  copyright2 : Subsystem
      mask Display:
      | text(10,90,'MLIB_Mnac_BAM_F16.mdl');text(10,75,'Multiply-negative-accumulate.');text(10,60,'Freescale')
      | text(10,45,'1.0');text(10,30,'27-Mar-2015');
  logo : Subsystem
      mask Display: image(imread('logo.jpg'))
  f16Out : Outport
  wires:
  MLIB_Mnac_SF/1 -> f16Out/1
  f16In3/1 -> MLIB_Mnac_SF/3
  f16In2/1 -> MLIB_Mnac_SF/2
  f16In1/1 -> MLIB_Mnac_SF/1

== system ammclib_bam_s32k14x/MLIB/bam_f16/MLIB_Msu_F16 ==
  note: ---------------------------------------------------------------------------------------------------------------------------------------------------------------------------------------------------
  f16In1 : Inport
  f16In2 : Inport  Port=2
  f16In3 : Inport  Port=3
  MLIB_Msu_SF : S-Function  FunctionName=MLIB_Msu_SF_F16  SFunctionDeploymentMode=off  EnableBusSupport=off
  copyright : Subsystem
      mask Display:
      | text(10,90,'FILE:');text(10,75,'DESRIPTION:')
      | text(10,60,'COPYRIGHT:')
      | text(10,45,'VERSION:')
      | text(10,30,'DATE:')
  copyright2 : Subsystem
      mask Display:
      | text(10,90,'MLIB_Msu_BAM_F16.mdl');text(10,75,'Multiply-subtract-from.');text(10,60,'NXP')
      | text(10,45,'1.0');text(10,30,'27-Mar-2015');
  logo : Subsystem
      mask Display: image(imread('logo.jpg'))
  f16Out : Outport
  wires:
  MLIB_Msu_SF/1 -> f16Out/1
  f16In3/1 -> MLIB_Msu_SF/3
  f16In2/1 -> MLIB_Msu_SF/2
  f16In1/1 -> MLIB_Msu_SF/1

== system ammclib_bam_s32k14x/MLIB/bam_f16/MLIB_MulSat_F16 ==
  note: ---------------------------------------------------------------------------------------------------------------------------------------------------------------------------------------------------
  f16In1 : Inport
  f16In2 : Inport  Port=2
  MLIB_MulSat_SF : S-Function  FunctionName=MLIB_MulSat_SF_F16  SFunctionDeploymentMode=off  EnableBusSupport=off
  copyright : Subsystem
      mask Display:
      | text(10,90,'FILE:');text(10,75,'DESRIPTION:')
      | text(10,60,'COPYRIGHT:')
      | text(10,45,'VERSION:')
      | text(10,30,'DATE:')
  copyright2 : Subsystem
      mask Display:
      | text(10,90,'MLIB_MulSat_BAM_F16.mdl');text(10,75,'Saturated sum of two input values.');text(10,60,'NXP')
      | text(10,45,'0.1');text(10,30,'01-Aug-2011');
  logo : Subsystem
      mask Display: image(imread('logo.jpg'))
  f16Out : Outport
  wires:
  MLIB_MulSat_SF/1 -> f16Out/1
  f16In2/1 -> MLIB_MulSat_SF/2
  f16In1/1 -> MLIB_MulSat_SF/1

== system ammclib_bam_s32k14x/MLIB/bam_f16/MLIB_Mul_F16 ==
  note: ---------------------------------------------------------------------------------------------------------------------------------------------------------------------------------------------------
  f16In1 : Inport
  f16In2 : Inport  Port=2
  MLIB_Mul_SF : S-Function  FunctionName=MLIB_Mul_SF_F16  SFunctionDeploymentMode=off  EnableBusSupport=off
  copyright : Subsystem
      mask Display:
      | text(10,90,'FILE:');text(10,75,'DESRIPTION:')
      | text(10,60,'COPYRIGHT:')
      | text(10,45,'VERSION:')
      | text(10,30,'DATE:')
  copyright2 : Subsystem
      mask Display:
      | text(10,90,'MLIB_Mul_BAM_F16.mdl');text(10,75,'Sum of two input values.');text(10,60,'NXP')
      | text(10,45,'0.1');text(10,30,'26-Jul-2011');
  logo : Subsystem
      mask Display: image(imread('logo.jpg'))
  f16Out : Outport
  wires:
  MLIB_Mul_SF/1 -> f16Out/1
  f16In2/1 -> MLIB_Mul_SF/2
  f16In1/1 -> MLIB_Mul_SF/1

== system ammclib_bam_s32k14x/MLIB/bam_f16/MLIB_NegSat_F16 ==
  note: ---------------------------------------------------------------------------------------------------------------------------------------------------------------------------------------------------
  f16In : Inport
  MLIB_NegSat_SF : S-Function  FunctionName=MLIB_NegSat_SF_F16  SFunctionDeploymentMode=off  EnableBusSupport=off
  copyright : Subsystem
      mask Display:
      | text(10,90,'FILE:');text(10,75,'DESRIPTION:')
      | text(10,60,'COPYRIGHT:')
      | text(10,45,'VERSION:')
      | text(10,30,'DATE:')
  copyright2 : Subsystem
      mask Display:
      | text(10,90,'MLIB_NegSat_BAM_F16.mdl');text(10,75,'Sum of two input values.');text(10,60,'NXP')
      | text(10,45,'0.1');text(10,30,'12-Jul-2011');
  logo : Subsystem
      mask Display: image(imread('logo.jpg'))
  f16Out : Outport
  wires:
  MLIB_NegSat_SF/1 -> f16Out/1
  f16In/1 -> MLIB_NegSat_SF/1

== system ammclib_bam_s32k14x/MLIB/bam_f16/MLIB_Neg_F16 ==
  note: ---------------------------------------------------------------------------------------------------------------------------------------------------------------------------------------------------
  f16In : Inport
  MLIB_Neg_SF : S-Function  FunctionName=MLIB_Neg_SF_F16  SFunctionDeploymentMode=off  EnableBusSupport=off
  copyright : Subsystem
      mask Display:
      | text(10,90,'FILE:');text(10,75,'DESRIPTION:')
      | text(10,60,'COPYRIGHT:')
      | text(10,45,'VERSION:')
      | text(10,30,'DATE:')
  copyright2 : Subsystem
      mask Display:
      | text(10,90,'MLIB_Neg_BAM_F16.mdl');text(10,75,'Sum of two input values.');text(10,60,'NXP')
      | text(10,45,'0.1');text(10,30,'20-Jan-2012');
  logo : Subsystem
      mask Display: image(imread('logo.jpg'))
  f16Out : Outport
  wires:
  MLIB_Neg_SF/1 -> f16Out/1
  f16In/1 -> MLIB_Neg_SF/1

== system ammclib_bam_s32k14x/MLIB/bam_f16/MLIB_Norm_F16 ==
  note: ---------------------------------------------------------------------------------------------------------------------------------------------------------------------------------------------------
  f16In : Inport
  MLIB_Norm_SF_F16 : S-Function  FunctionName=MLIB_Norm_SF_F16  SFunctionDeploymentMode=off  EnableBusSupport=off
  copyright : Subsystem
      mask Display:
      | text(10,90,'FILE:');text(10,75,'DESRIPTION:')
      | text(10,60,'COPYRIGHT:')
      | text(10,45,'VERSION:')
      | text(10,30,'DATE:')
  copyright2 : Subsystem
      mask Display:
      | text(10,90,'MLIB_Norm_BAM_F16.mdl');text(10,75,'Normalization of the input value.');text(10,60,'Freescale')
      | text(10,45,'0.1');text(10,30,'15-Sep-2011');
  logo : Subsystem
      mask Display: image(imread('logo.jpg'))
  u16Out : Outport
  wires:
  MLIB_Norm_SF_F16/1 -> u16Out/1
  f16In/1 -> MLIB_Norm_SF_F16/1

== system ammclib_bam_s32k14x/MLIB/bam_f16/MLIB_RndSat_F16F32 ==
  note: ---------------------------------------------------------------------------------------------------------------------------------------------------------------------------------------------------
  f32In : Inport
  MLIB_RndSat_SF : S-Function  FunctionName=MLIB_RndSat_SF_F16F32  SFunctionDeploymentMode=off  EnableBusSupport=off
  copyright : Subsystem
      mask Display: text(10,90,'FILE:');text(10,75,'DESRIPTION:');text(10,60,'COPYRIGHT:');text(10,45,'VERSION:');text(10,30,'DATE:')
  copyright2 : Subsystem
      mask Display: text(10,90,'MLIB_RndSat_BAM_F16F32.mdl');text(10,75,'Rounding of the input value to the nearest saturated value in output format.');text(10,60,'NXP');text(10,45,'1.0');text(10,30,'05-May-2016');
  logo : Subsystem
      mask Display: image(imread('logo.jpg'))
  f16Out : Outport
  wires:
  MLIB_RndSat_SF/1 -> f16Out/1
  f32In/1 -> MLIB_RndSat_SF/1

== system ammclib_bam_s32k14x/MLIB/bam_f16/MLIB_Round_F16 ==
  note: ---------------------------------------------------------------------------------------------------------------------------------------------------------------------------------------------------
  f16In1 : Inport
  u16In2 : Inport  Port=2
  MLIB_Round_SF_F16 : S-Function  FunctionName=MLIB_Round_SF_F16  SFunctionDeploymentMode=off  EnableBusSupport=off
  copyright : Subsystem
      mask Display:
      | text(10,90,'FILE:');text(10,75,'DESRIPTION:')
      | text(10,60,'COPYRIGHT:')
      | text(10,45,'VERSION:')
      | text(10,30,'DATE:')
  copyright2 : Subsystem
      mask Display:
      | text(10,90,'MLIB_Round_BAM_F16.mdl');text(10,75,'Round the first input value.');text(10,60,'Freescale')
      | text(10,45,'0.1');text(10,30,'02-Sep-2011');
  logo : Subsystem
      mask Display: image(imread('logo.jpg'))
  f16Out : Outport
  wires:
  MLIB_Round_SF_F16/1 -> f16Out/1
  u16In2/1 -> MLIB_Round_SF_F16/2
  f16In1/1 -> MLIB_Round_SF_F16/1

== system ammclib_bam_s32k14x/MLIB/bam_f16/MLIB_ShBiSat_F16 ==
  note: ---------------------------------------------------------------------------------------------------------------------------------------------------------------------------------------------------
  f16In1 : Inport
  s16In2 : Inport  Port=2
  MLIB_ShBiSat_SF_F16 : S-Function  FunctionName=MLIB_ShBiSat_SF_F16  SFunctionDeploymentMode=off  EnableBusSupport=off
  copyright : Subsystem
      mask Display:
      | text(10,90,'FILE:');text(10,75,'DESRIPTION:')
      | text(10,60,'COPYRIGHT:')
      | text(10,45,'VERSION:')
      | text(10,30,'DATE:')
  copyright2 : Subsystem
      mask Display:
      | text(10,90,'MLIB_ShBiSat_BAM_F16.mdl');text(10,75,'Shift the first parameter to left or right and saturate if necessary.');text(10,60,'NXP')
      | text(10,45,'0.1');text(10,30,'26-Aug-2011');
  logo : Subsystem
      mask Display: image(imread('logo.jpg'))
  f16Out : Outport
  wires:
  MLIB_ShBiSat_SF_F16/1 -> f16Out/1
  s16In2/1 -> MLIB_ShBiSat_SF_F16/2
  f16In1/1 -> MLIB_ShBiSat_SF_F16/1

== system ammclib_bam_s32k14x/MLIB/bam_f16/MLIB_ShBi_F16 ==
  note: ---------------------------------------------------------------------------------------------------------------------------------------------------------------------------------------------------
  f16In1 : Inport
  s16In2 : Inport  Port=2
  MLIB_ShBi_SF_F16 : S-Function  FunctionName=MLIB_ShBi_SF_F16  SFunctionDeploymentMode=off  EnableBusSupport=off
  copyright : Subsystem
      mask Display:
      | text(10,90,'FILE:');text(10,75,'DESRIPTION:')
      | text(10,60,'COPYRIGHT:')
      | text(10,45,'VERSION:')
      | text(10,30,'DATE:')
  copyright2 : Subsystem
      mask Display:
      | text(10,90,'MLIB_ShBi_BAM_F16.mdl');text(10,75,'Shift the first parameter to left or right.');text(10,60,'NXP')
      | text(10,45,'0.1');text(10,30,'24-Aug-2011');
  logo : Subsystem
      mask Display: image(imread('logo.jpg'))
  f16Out : Outport
  wires:
  MLIB_ShBi_SF_F16/1 -> f16Out/1
  s16In2/1 -> MLIB_ShBi_SF_F16/2
  f16In1/1 -> MLIB_ShBi_SF_F16/1

== system ammclib_bam_s32k14x/MLIB/bam_f16/MLIB_ShLSat_F16 ==
  note: ---------------------------------------------------------------------------------------------------------------------------------------------------------------------------------------------------
  f16In1 : Inport
  u16In2 : Inport  Port=2
  MLIB_ShLSat_SF : S-Function  FunctionName=MLIB_ShLSat_SF_F16  SFunctionDeploymentMode=off  EnableBusSupport=off
  copyright : Subsystem
      mask Display:
      | text(10,90,'FILE:');text(10,75,'DESRIPTION:')
      | text(10,60,'COPYRIGHT:')
      | text(10,45,'VERSION:')
      | text(10,30,'DATE:')
  copyright2 : Subsystem
      mask Display:
      | text(10,90,'MLIB_ShLSat_BAM_F16.mdl');text(10,75,'Shift the first parameter to left and saturate if necessary.');text(10,60,'NXP')
      | text(10,45,'0.1');text(10,30,'19-Jul-2011');
  logo : Subsystem
      mask Display: image(imread('logo.jpg'))
  f16Out : Outport
  wires:
  MLIB_ShLSat_SF/1 -> f16Out/1
  u16In2/1 -> MLIB_ShLSat_SF/2
  f16In1/1 -> MLIB_ShLSat_SF/1

== system ammclib_bam_s32k14x/MLIB/bam_f16/MLIB_ShL_F16 ==
  note: ---------------------------------------------------------------------------------------------------------------------------------------------------------------------------------------------------
  f16In1 : Inport
  u16In2 : Inport  Port=2
  MLIB_ShL_SF_F16 : S-Function  FunctionName=MLIB_ShL_SF_F16  SFunctionDeploymentMode=off  EnableBusSupport=off
  copyright : Subsystem
      mask Display:
      | text(10,90,'FILE:');text(10,75,'DESRIPTION:')
      | text(10,60,'COPYRIGHT:')
      | text(10,45,'VERSION:')
      | text(10,30,'DATE:')
      | text(10,15,'AUTHOR:')
  copyright2 : Subsystem
      mask Display:
      | text(10,90,'MLIB_ShL_BAM_F16.mdl');text(10,75,'Shift the first parameter to left.');text(10,60,'Freescale')
      | text(10,45,'0.1');text(10,30,'04-Jul-2011');text(10,15,'');
  logo : Subsystem
      mask Display: image(imread('logo.jpg'))
  f16Out : Outport
  wires:
  u16In2/1 -> MLIB_ShL_SF_F16/2
  MLIB_ShL_SF_F16/1 -> f16Out/1
  f16In1/1 -> MLIB_ShL_SF_F16/1

== system ammclib_bam_s32k14x/MLIB/bam_f16/MLIB_ShR_F16 ==
  note: ---------------------------------------------------------------------------------------------------------------------------------------------------------------------------------------------------
  f16In1 : Inport
  u16In2 : Inport  Port=2
  MLIB_ShR_SF : S-Function  FunctionName=MLIB_ShR_SF_F16  SFunctionDeploymentMode=off  EnableBusSupport=off
  copyright : Subsystem
      mask Display:
      | text(10,90,'FILE:');text(10,75,'DESRIPTION:')
      | text(10,60,'COPYRIGHT:')
      | text(10,45,'VERSION:')
      | text(10,30,'DATE:')
  copyright2 : Subsystem
      mask Display:
      | text(10,90,'MLIB_ShR_BAM_F16.mdl');text(10,75,'Shift the first parameter to right.');text(10,60,'Freescale')
      | text(10,45,'0.1');text(10,30,'20-Jul-2011');
  logo : Subsystem
      mask Display: image(imread('logo.jpg'))
  f16Out : Outport
  wires:
  MLIB_ShR_SF/1 -> f16Out/1
  u16In2/1 -> MLIB_ShR_SF/2
  f16In1/1 -> MLIB_ShR_SF/1

== system ammclib_bam_s32k14x/MLIB/bam_f16/MLIB_SubSat_F16 ==
  note: ---------------------------------------------------------------------------------------------------------------------------------------------------------------------------------------------------
  f16In1 : Inport
  f16In2 : Inport  Port=2
  MLIB_SubSat_SF : S-Function  FunctionName=MLIB_SubSat_SF_F16  SFunctionDeploymentMode=off  EnableBusSupport=off
  copyright : Subsystem
      mask Display:
      | text(10,90,'FILE:');text(10,75,'DESRIPTION:')
      | text(10,60,'COPYRIGHT:')
      | text(10,45,'VERSION:')
      | text(10,30,'DATE:')
  copyright2 : Subsystem
      mask Display:
      | text(10,90,'MLIB_SubSat_BAM_F16.mdl');text(10,75,'Saturated sum of two input values.');text(10,60,'NXP')
      | text(10,45,'0.1');text(10,30,'20-Jan-2012');
  logo : Subsystem
      mask Display: image(imread('logo.jpg'))
  f16Out : Outport
  wires:
  MLIB_SubSat_SF/1 -> f16Out/1
  f16In2/1 -> MLIB_SubSat_SF/2
  f16In1/1 -> MLIB_SubSat_SF/1
